simulink model "ssc_Probes_test_all_16b"  (R2019b)
(part 2 of 4)

      | set_param(gcb, 'AttributesFormatString', strcat('[', unit,']'));
      mask help: Simscape Probe
      settings: AttributesFormatString=[K]
      settings: CopyFcn=|
      | set_param(gcb,'LinkStatus','inactive');
      | set_param(gcb,'LinkStatus','none');
      | set_param([gcb '/Goto'],'GotoTag', [get(gcbh,'name')]);
      | set_param([gcb '/From'],'GotoTag', [get(gcbh,'name')]);
      | h = get_param([gcb, '/PS-S'], 'PortHandles');
      | set(h.Outport(1), 'SignalNameFromLabel', [get(gcbh,'name')])
      | clear h;
      settings: NameChangeFcn=|
      | set_param([gcb '/Goto'],'GotoTag', [get(gcbh,'name')]);
      | set_param([gcb '/From'],'GotoTag', [get(gcbh,'name')]);
      | h = get_param([gcb, '/PS-S'], 'PortHandles');
      | set(h.Outport(1), 'SignalNameFromLabel', [get(gcbh,'name')])
      | clear h;
      settings: OpenFcn=|
      | if exist('logsout', 'var')
      |   vname = get(gcbh,'name');
      |   fHandle = findall(0,'Tag',vname);
      |   if isempty(fHandle)
      |   figure('Tag',vname);
      |   end;
      |   figure(findobj('Tag',vname));
      |   plot(logsout.getElement([gcb, '/PS-S'], '-blockpath').Values)
      |   title(get(gcbh,'name'));
      |   ylabel(['Temperature (' get_param([gcb '/PS-S'],'Unit') ')'] );
      | end
      mask Display:
      | port_label('RConn', 1,'-');
      | port_label('LConn', 1,'+');
  dTemperature_TL : Subsystem  Description=Simscape Probe  InitFcn=|
      | unit=get_param([gcb '/PS-S'],'Unit');                                              
      | set_param(gcb, 'AttributesFormatString', strcat('[', unit,']'));
      mask help: Simscape Probe
      settings: AttributesFormatString=[K]
      settings: CopyFcn=|
      | set_param(gcb,'LinkStatus','inactive');
      | set_param(gcb,'LinkStatus','none');
      | set_param([gcb '/Goto'],'GotoTag', [get(gcbh,'name')]);
      | set_param([gcb '/From'],'GotoTag', [get(gcbh,'name')]);
      | h = get_param([gcb, '/PS-S'], 'PortHandles');
      | set(h.Outport(1), 'SignalNameFromLabel', [get(gcbh,'name')])
      | clear h;
      settings: NameChangeFcn=|
      | set_param([gcb '/Goto'],'GotoTag', [get(gcbh,'name')]);
      | set_param([gcb '/From'],'GotoTag', [get(gcbh,'name')]);
      | h = get_param([gcb, '/PS-S'], 'PortHandles');
      | set(h.Outport(1), 'SignalNameFromLabel', [get(gcbh,'name')])
      | clear h;
      settings: OpenFcn=|
      | if exist('logsout', 'var')
      |   vname = get(gcbh,'name');
      |   fHandle = findall(0,'Tag',vname);
      |   if isempty(fHandle)
      |   figure('Tag',vname);
      |   end;
      |   figure(findobj('Tag',vname));
      |   plot(logsout.getElement([gcb, '/PS-S'], '-blockpath').Values)
      |   title(get(gcbh,'name'));
      |   ylabel(['Temperature (' get_param([gcb '/PS-S'],'Unit') ')'] );
      | end
      mask Display:
      | port_label('RConn', 1,'-');
      | port_label('LConn', 1,'+');
  dVelocity : Subsystem  Description=Simscape Probe  InitFcn=|
      | unit=get_param([gcb '/PS-S'],'Unit');                                              
      | set_param(gcb, 'AttributesFormatString', strcat('[', unit,']'));
      mask help: Simscape Probe
      settings: AttributesFormatString=[m/s]
      settings: CopyFcn=|
      | set_param(gcb,'LinkStatus','inactive');
      | set_param(gcb,'LinkStatus','none');
      | set_param([gcb '/Goto'],'GotoTag', [get(gcbh,'name')]);
      | set_param([gcb '/From'],'GotoTag', [get(gcbh,'name')]);
      | h = get_param([gcb, '/PS-S'], 'PortHandles');
      | set(h.Outport(1), 'SignalNameFromLabel', [get(gcbh,'name')])
      | clear h;
      settings: NameChangeFcn=|
      | set_param([gcb '/Goto'],'GotoTag', [get(gcbh,'name')]);
      | set_param([gcb '/From'],'GotoTag', [get(gcbh,'name')]);
      | h = get_param([gcb, '/PS-S'], 'PortHandles');
      | set(h.Outport(1), 'SignalNameFromLabel', [get(gcbh,'name')])
      | clear h;
      settings: OpenFcn=|
      | if exist('logsout', 'var')
      |   vname = get(gcbh,'name');
      |   fHandle = findall(0,'Tag',vname);
      |   if isempty(fHandle)
      |   figure('Tag',vname);
      |   end;
      |   figure(findobj('Tag',vname));
      |   plot(logsout.getElement([gcb, '/PS-S'], '-blockpath').Values)
      |   title(get(gcbh,'name'));
      |   ylabel(['Velocity (' get_param([gcb '/PS-S'],'Unit') ')'] );
      | end
      mask Display:
      | port_label('RConn', 1,'-');
      | port_label('LConn', 1,'+');
  dVoltage : Subsystem  Description=Simscape Probe  InitFcn=|
      | unit=get_param([gcb '/PS-S'],'Unit');                                              
      | set_param(gcb, 'AttributesFormatString', strcat('[', unit,']'));
      mask help: Simscape Probe
      settings: AttributesFormatString=[V]
      settings: CopyFcn=|
      | set_param(gcb,'LinkStatus','inactive');
      | set_param(gcb,'LinkStatus','none');
      | set_param([gcb '/Goto'],'GotoTag', [get(gcbh,'name')]);
      | set_param([gcb '/From'],'GotoTag', [get(gcbh,'name')]);
      | h = get_param([gcb, '/PS-S'], 'PortHandles');
      | set(h.Outport(1), 'SignalNameFromLabel', [get(gcbh,'name')])
      | clear h;
      settings: NameChangeFcn=|
      | set_param([gcb '/Goto'],'GotoTag', [get(gcbh,'name')]);
      | set_param([gcb '/From'],'GotoTag', [get(gcbh,'name')]);
      | h = get_param([gcb, '/PS-S'], 'PortHandles');
      | set(h.Outport(1), 'SignalNameFromLabel', [get(gcbh,'name')])
      | clear h;
      settings: OpenFcn=|
      | if exist('logsout', 'var')
      |   vname = get(gcbh,'name');
      |   fHandle = findall(0,'Tag',vname);
      |   if isempty(fHandle)
      |   figure('Tag',vname);
      |   end;
      |   figure(findobj('Tag',vname));
      |   plot(logsout.getElement([gcb, '/PS-S'], '-blockpath').Values)
      |   title(get(gcbh,'name'));
      |   ylabel(['Voltage (' get_param([gcb '/PS-S'],'Unit') ')'] );
      | end
      mask Display:
      | port_label('RConn', 1,'-');
      | port_label('LConn', 1,'+');
  wires:
  Sine Wave/1 -> Simulink-PS Converter/1
  Sine Wave1/1 -> Simulink-PS Converter1/1
  Sine Wave2/1 -> Simulink-PS Converter2/1
  Sine Wave3/1 -> Simulink-PS Converter3/1
  Sine Wave4/1 -> Simulink-PS Converter4/1
  Sine Wave5/1 -> Simulink-PS Converter5/1
  Sine Wave7/1 -> Simulink-PS Converter7/1
  Sine Wave6/1 -> Gain/1
  Gain/1 -> Simulink-PS Converter6/1
  Sine Wave8/1 -> Simulink-PS Converter8/1
  connections:
  Controlled Voltage Source/RConn1 -- Simulink-PS Converter/RConn1
  Electrical Reference/LConn1 -- Solver Configuration/RConn1 -- dVoltage/RConn1 -- Resistor/RConn1 -- Controlled Voltage Source/RConn2
  Current/LConn1 -- Controlled Voltage Source/LConn1
  Controlled MMF Source/RConn1 -- Simulink-PS Converter1/RConn1
  Reluctance/LConn1 -- Flux/RConn1 -- MMF/LConn1 -- dMMF/LConn1
  Flux/LConn1 -- Controlled MMF Source/LConn1
  Magnetic Reference/LConn1 -- Solver Configuration1/RConn1 -- dMMF/RConn1 -- Reluctance/RConn1 -- Controlled MMF Source/RConn2
  Force/LConn1 -- Ideal Force Source/LConn1
  Mass/LConn1 -- Force/RConn1 -- Velocity/LConn1 -- Translational Spring/LConn1 -- dVelocity/LConn1 -- Position/LConn1 -- dPosition/LConn1
  Mechanical Translational Reference/LConn1 -- Solver Configuration2/RConn1 -- Ideal Force Source/RConn2 -- dPosition/RConn1 -- dVelocity/RConn1 -- Translational Spring/RConn1
  Ideal Force Source/RConn1 -- Simulink-PS Converter2/RConn1
  Simulink-PS Converter3/RConn1 -- Ideal Torque Source/RConn1
  Solver Configuration3/RConn1 -- Mechanical Rotational Reference/LConn1 -- dAngle/RConn1 -- dAngVel/RConn1 -- Rotational Spring/RConn1 -- Ideal Torque Source/RConn2
  Torque/LConn1 -- Ideal Torque Source/LConn1
  Inertia/LConn1 -- Torque/RConn1 -- AngVel/LConn1 -- dAngVel/LConn1 -- Angle/LConn1 -- dAngle/LConn1 -- Rotational Spring/LConn1
  Simulink-PS Converter4/RConn1 -- Hydraulic Pressure Source/RConn1
  Hydraulic Reference/LConn1 -- Solver Configuration4/RConn1 -- dPressure/RConn1 -- Constant Area Hydraulic Orifice/RConn1 -- Hydraulic Pressure Source/RConn2
  Flow/LConn1 -- Hydraulic Pressure Source/LConn1
  Pressure/LConn1 -- dPressure/LConn1 -- Flow/RConn1 -- Constant Area Hydraulic Orifice/LConn1
  HeatFlow/LConn1 -- Ideal Heat Flow Source/LConn1
  Temperature/LConn1 -- dTemperature/LConn1 -- HeatFlow/RConn1 -- Conductive Heat Transfer/LConn1
  Simulink-PS Converter5/RConn1 -- Ideal Heat Flow Source/RConn1
  Solver Configuration5/RConn1 -- dTemperature/RConn1 -- Conductive Heat Transfer/RConn1 -- Ideal Heat Flow Source/RConn2 -- Thermal Reference/LConn1
  Pneumatic Absolute Reference/LConn1 -- Gas Properties/RConn1 -- Solver Configuration6/RConn1 -- Pneumatic Resistive Tube1/RConn1 -- dGasTemperature/RConn1 -- dGasPressure/RConn1 -- Controlled Pneumatic Pressure Source/RConn1
  Controlled Pneumatic Pressure Source/RConn2 -- Simulink-PS Converter6/RConn1
  Controlled Pneumatic Pressure Source/LConn1 -- MassFlow/LConn1
  GasHeatFlow/LConn1 -- MassFlow/RConn1
  Resistor/LConn1 -- Current/RConn1 -- Voltage/LConn1 -- dVoltage/LConn1
  Repeating Sequence/RConn1 -- PhysicalSignal/LConn1 -- Solver Configuration7/RConn1
  AbsTemperature_TL/LConn1 -- AbsPressure_TL/LConn1 -- ThermalFlux_TL/RConn1 -- dTemperature_TL/LConn1 -- dPressure_TL/LConn1 -- Local Restriction (TL)/LConn1
  ThermalFlux_TL/LConn1 -- MassFlow_TL/RConn1
  MassFlow_TL/LConn1 -- Controlled Pressure Source (TL)/RConn1
  Controlled Pressure Source (TL)/LConn2 -- Simulink-PS Converter7/RConn1
  Solver Configuration8/RConn1 -- dTemperature_TL/RConn1 -- dPressure_TL/RConn1 -- Local Restriction (TL)/RConn1 -- Temperature Reservoir (TL)/LConn1 -- Controlled Pressure Source (TL)/LConn1
  AtmTemperature/LConn1 -- dGasTemperature/LConn1 -- dGasPressure/LConn1 -- GasHeatFlow/RConn1 -- Pneumatic Resistive Tube1/LConn1 -- AbsTemperature/LConn1 -- AbsPressure/LConn1 -- GaugePressure/LConn1
  AbsPressure_2P/LConn1 -- InternalEnergy_2P/LConn1 -- Translational Mechanical Converter (2P)/LConn1 -- VolumetricFlow_2P/RConn1
  Translational Damper/LConn1 -- Translational Mechanical Converter (2P)/RConn1 -- Mass1/LConn1
  Controlled Pressure Source (2P)/LConn1 -- Two-Phase Fluid Properties (2P)/RConn1 -- Reservoir (2P)/LConn1 -- Solver Configuration9/RConn1
  Controlled Pressure Source (2P)/RConn1 -- dEnergy_2P/LConn1 -- dPressure_2P/LConn1 -- Local Restriction (2P)/LConn1
  Translational Mechanical Converter (2P)/LConn3 -- Perfect Insulator/LConn1
  Simulink-PS Converter8/RConn1 -- Controlled Pressure Source (2P)/LConn2
  Mechanical Translational Reference2/LConn1 -- Translational Damper/RConn1
  Translational Mechanical Converter (2P)/LConn2 -- Mechanical Translational Reference1/LConn1
  Local Restriction (2P)/RConn1 -- MassFlow_2P/LConn1 -- dEnergy_2P/RConn1 -- dPressure_2P/RConn1
  AbsTemp_2P/LConn1 -- SpecificVol_2P/LConn1 -- VaporMassFraction_2P/LConn1 -- Enthalpy_2P/LConn1 -- ThermoProps_2P/LConn1 -- MassFlow_2P/RConn1 -- EnergyFlow_2P/LConn1
  VolumetricFlow_2P/LConn1 -- EnergyFlow_2P/RConn1
